simulink model "kalman_tank_based_fv"  (R2020b)
settings: Solver=ode45  StartTime=0.0  StopTime=30  RelTol=1e-3
values from neighbouring files (symbols this model uses):
  A = [1 Ts ... (first row only)    [kalman_hw7_main_fv.m]
  alpha = 0.5    [kalman_hw7_main_fv.m]
  Amp = 0.8    [kalman_hw7_main_fv.m]
  Be = 20    [kalman_hw7_main_fv.m]
  beta = 0.01    [kalman_hw7_main_fv.m]
  Bh = 1.5    [kalman_hw7_main_fv.m]
  Bs = 50    [kalman_hw7_main_fv.m]
  C = [1 0]    [kalman_hw7_main_fv.m]
  delay = 10    [kalman_hw7_main_fv.m]
  Dh = 2    [kalman_hw7_main_fv.m]
  Dm = 0    [kalman_hw7_main_fv.m]
  Ds = 0    [kalman_hw7_main_fv.m]
  Fc_lp = 5    [kalman_hw7_main_fv.m]
  Fc_sin = 0.1    [kalman_hw7_main_fv.m]
  H0_m = 1    [kalman_hw7_main_fv.m]
  H0_s = 1    [kalman_hw7_main_fv.m]
  H_D = 0.5    [kalman_hw7_main_fv.m]
  Je = 0    [kalman_hw7_main_fv.m]
  Jh = 0    [kalman_hw7_main_fv.m]
  Ke = 210    [kalman_hw7_main_fv.m]
  Kh = 0.1    [kalman_hw7_main_fv.m]
  Ks = 40    [kalman_hw7_main_fv.m]
  Mm = 0.5    [kalman_hw7_main_fv.m]
  Ms = 2    [kalman_hw7_main_fv.m]
  Ph = 1    [kalman_hw7_main_fv.m]
  posNoiseVar = 0.001    [kalman_hw7_main_fv.m]
  R_m = 1    [kalman_hw7_main_fv.m]
  R_s = 1    [kalman_hw7_main_fv.m]
  torqueNoiseVar = 0.001    [kalman_hw7_main_fv.m]
  Ts = 0.001    [kalman_hw7_main_fv.m]
  xe = 0.5    [kalman_hw7_main_fv.m]
undefined symbols (not defined in the file or in its folder): Discrete, Time
libraries: simulink x2, ctrlSharedLib x2
settings Model: Creator=nicol  LastModifiedBy=nicol

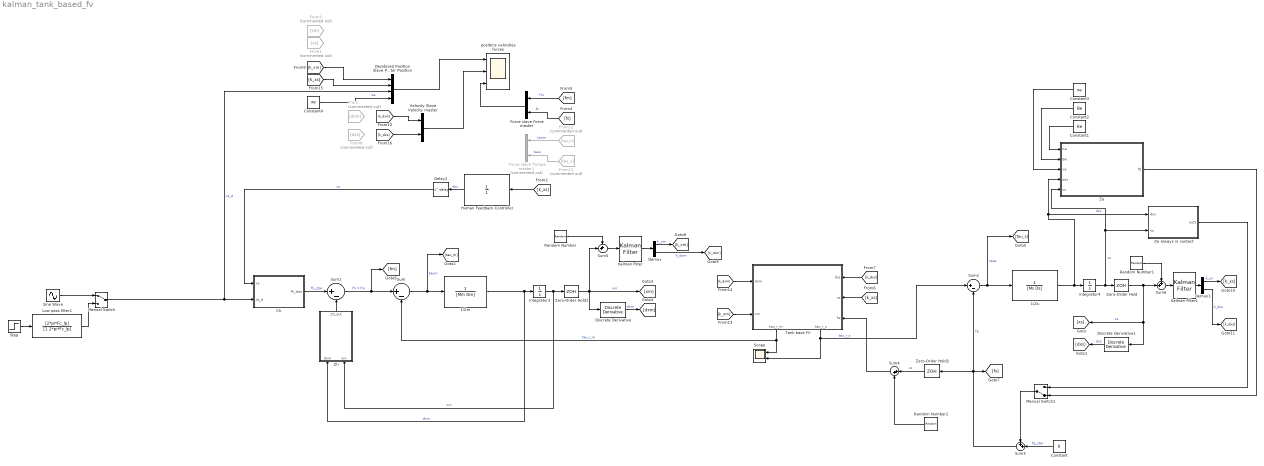
== system kalman_tank_based_fv ==
  1/Zm : TransferFcn  Denominator=[Mm Dm]
  1/Zs : TransferFcn  Denominator=[Ms Ds]
  Ch : Subsystem
  Constant : Constant  Value=0
  Constant1 : Constant  Value=Ke
  Constant2 : Constant  Value=Be
  Constant3 : Constant  Value=xe
  Constant4 : Constant  Value=xe
  Delay2 : Delay  DelayLength=delay  SampleTime=Ts
  Demux : Demux  Outputs=2
  Demux1 : Demux  Outputs=2
  Desidered Position Slave Position Master Position : Mux
  Discrete Derivative : simulink/Discrete/Discrete Derivative  gainval=1.0  ICPrevScaledInput=0.0  OutMin=[]  OutMax=[]  OutDataType=fixdt(1, 16)  OutScaling=2^-10  DoSatur=off
  Discrete Derivative1 : simulink/Discrete/Discrete Derivative  gainval=1.0  ICPrevScaledInput=0.0  OutMin=[]  OutMax=[]  OutDataType=fixdt(1, 16)  OutScaling=2^-10  DoSatur=off
  Force slave Force master : Mux  Inputs=2
  From : From  Commented=on  GotoTag=dxm
  From1 : From  Commented=on  GotoTag=xs
  From11 : From  Commented=on  GotoTag=tau_s
  From12 : From  Commented=on  GotoTag=tau_m
  From3 : From  Commented=on  GotoTag=xm
  From8 : From  Commented=on  GotoTag=dxs
  Human Feedback Controller : TransferFcn  Denominator=[1]
  Integrator3 : Integrator
  Integrator4 : Integrator
  Kalman Filter : ctrlSharedLib/Kalman Filter  TimeDomain=Discrete-Time  UseCurrentEstimator=on  ModelSource=Individual A, B, C, D matrices  ModelSourceVariable=ss(0.95,1,0,0,Ts)  A=A  B=1  C=C  D=0  NumberOfStates=1  NumberOfInputs=1  NumberOfOutputs=1  InitialEstimateSource=Dialog  X0=0  P0=10  UseK=off  UseGH=off  NumberOfProcessNoiseInputs=1  G=1  TimeInvariantG=on  H=0  TimeInvariantH=on  Q=Q_m  TimeInvariantQ=on  R=R_m  TimeInvariantR=on  N=0  TimeInvariantN=on  AddInputPort=off  AddEnablePort=off  OutputEstimatedY=off  OutputP=off  Ts=Ts
  Kalman Filter1 : ctrlSharedLib/Kalman Filter  TimeDomain=Discrete-Time  UseCurrentEstimator=on  ModelSource=Individual A, B, C, D matrices  ModelSourceVariable=ss(0.95,1,0,0,Ts)  A=A  B=1  C=C  D=0  NumberOfStates=1  NumberOfInputs=1  NumberOfOutputs=1  InitialEstimateSource=Dialog  X0=0  P0=10  UseK=off  UseGH=off  NumberOfProcessNoiseInputs=1  G=1  TimeInvariantG=on  H=0  TimeInvariantH=on  Q=Q_s  TimeInvariantQ=on  R=R_s  TimeInvariantR=on  N=0  TimeInvariantN=on  AddInputPort=off  AddEnablePort=off  OutputEstimatedY=off  OutputP=off  Ts=Ts
  Low pass filter1 : TransferFcn  Numerator=[2*pi*Fc_lp]  Denominator=[1 2*pi*Fc_lp]
  Manual Switch : ManualSwitch
  Manual Switch1 : ManualSwitch  CurrentSetting=0
  Random Number : RandomNumber  Variance=posNoiseVar  SampleTime=Ts
  Random Number1 : RandomNumber  Variance=posNoiseVar  SampleTime=Ts
  Random Number2 : RandomNumber  Variance=torqueNoiseVar  SampleTime=Ts
  Scope : Scope  NumInputPorts=2
  Sine Wave : Sin  Amplitude=Amp  Frequency=2*pi*Fc_sin  SampleTime=0
  Step : Step  Time=Amp  After=Amp  SampleTime=0
  Sum : Sum  Inputs=|+-
  Sum1 : Sum  Inputs=|+-
  Sum2 : Sum  Inputs=|+-
  Sum3 : Sum  Inputs=++|
  Sum4 : Sum  Inputs=|++
  Sum5 : Sum  Inputs=++|
  Sum6 : Sum  Inputs=++|
  Tank base FV : Subsystem
      settings: PortSchema="{\"entries\":[{\"content\":{\"sides\":[{\"content\":{\"connectorIds\":[\"In1\",\"In2\"]},\"type\":\"ConnectorPlacement.EquallySpacedRectSide\",\"uuid\":\"3a964002-fb37-4a92-b745-35f358b8e187\"},{\"content\":{\"connectorIds\":[\"In3\",\"In4\",\"In5\"],\"side\":\"RIGHT\"},\"type\":\"ConnectorPlacement.EquallySpacedRectSide\",\"uuid\":\"6a0ade08-0aa0-46a3-9e09-c310668c505c\"},{\"content\":{\"connectorIds\":[],\"side\":\"TOP\"},\"type\":\"ConnectorPlacement.EquallySpacedRectSide\",\"uuid\":\"1dfd7bbc-8185-4b5f-95de-42c58388ee02\"},{\"content\":{\"connectorIds\":[\"Out1\",\"Out2\"],\"side\":\"BOTTOM\"},\"type\":\"ConnectorPlacement.EquallySpacedRectSide\",\"uuid\":\"8c57ed43-4006-4572-ac50-c9adf88e8601\"},{\"content\":{\"connectorIds\":[],\"side\":\"HIDDEN\"},\"type\":\"ConnectorPlacement.EquallySpacedRectSide\",\"uuid\":\"15175a08-ca5b-4167-ba1d-f2e8cd3d814b\"}]},\"type\":\"ConnectorPlacement.EquallySpacedConnector\",\"uuid\":\"2bd1e993-3bc7-4875-9b20-3fb59092d5ec\"}],\"packageUris\":[\"http://schema.mathworks.com/mf0/Connector/R2020b\"],\"version\":\"1.0\"}"
  Torue slave Torque master1 : Mux  Commented=on  Inputs=2
  Velocity Slave Velocity master : Mux  Inputs=2
  Ze : MATLAB Function  TreatAsAtomicUnit=on
  Ze always in contact : Subsystem
  Zero-Order Hold : ZeroOrderHold  SampleTime=Ts
  Zero-Order Hold1 : ZeroOrderHold  SampleTime=Ts
  Zero-Order Hold2 : ZeroOrderHold  SampleTime=Ts
  Zh : Subsystem
  "positons velocities forces " : Scope  NumInputPorts=3
  wires:
  Ch/1(fh_star) -> Sum1/1  "fh_star"
  Zh/1(Zh_out) -> Sum1/2
  1/Zm/1 -> Zh/1(dxm), Integrator3/1  "dxm"
  Sum1/1 -> Sum/1, [fm]  "fh = fm"
  1/Zs/1 -> Integrator4/1, Ze always in contact/1(dxs), Ze/4(dxs)  "dxs"
  Sum2/1 -> 1/Zs/1, [tau_s]  "taus"
  Ze/1(fE) -> Manual Switch1/2
  Sum3/1 -> Zero-Order Hold2/1, Sum2/2, [fs]  "fe"
  Constant/1 -> Sum3/2  "fe_star"
  Constant1/1 -> Ze/1(Ke)
  Constant2/1 -> Ze/2(Be)
  Constant3/1 -> Ze/3(xe)
  Integrator4/1 -> Zero-Order Hold/1, Ze/5(xs), Ze always in contact/2(xs)  "xs"
  Manual Switch1/1 -> Sum3/1
  Ze always in contact/1(out1) -> Manual Switch1/1
  Sum/1 -> [tau_m], 1/Zm/1  "taum"
  Velocity Slave Velocity master/1 -> "positons velocities forces "/2
  Desidered Position Slave Position Master Position/1 -> "positons velocities forces "/1
  Manual Switch/1 -> Ch/2(xs_d), Desidered Position Slave Position Master Position/3  "xs_d"
  Integrator3/1 -> Zero-Order Hold1/1, Zh/2(xm)  "xm"
  [k_xs] -> Human Feedback Controller/1
  Delay2/1 -> Ch/1(xs)  "xs"
  Human Feedback Controller/1 -> Delay2/1  "dxs"
  Sine Wave/1 -> Manual Switch/1
  [k_dxm] -> Velocity Slave Velocity master/1
  [k_xs] -> Desidered Position Slave Position Master Position/2
  [k_xm] -> Desidered Position Slave Position Master Position/1
  Constant4/1 -> Desidered Position Slave Position Master Position/4  "xe"
  Step/1 -> Low pass filter1/1
  [k_dxs] -> Velocity Slave Velocity master/2
  Low pass filter1/1 -> Manual Switch/2
  Force slave Force master/1 -> "positons velocities forces "/3
  [fm] -> Force slave Force master/1  "fm"
  [fs] -> Force slave Force master/2  "fs"
  [k_dxm] -> Tank base FV/1(dxm)
  [k_xm] -> Tank base FV/2(xm)
  [k_dxs] -> Tank base FV/3(dxs)
  [k_xs] -> Tank base FV/4(xs)
  Tank base FV/1(tau_r_m) -> Sum/2, Scope/1  "tau_r_m"
  Tank base FV/2(tau_r_s) -> Sum2/1, Scope/2  "tau_r_s"
  From12/1 -> Torue slave Torque master1/1  "taum"
  From11/1 -> Torue slave Torque master1/2  "taus"
  Zero-Order Hold2/1 -> Sum4/1  "xs"
  Sum5/1 -> Kalman Filter/1
  Demux/1 -> [k_xm]  "k_xm"
  Random Number/1 -> Sum5/1
  Zero-Order Hold1/1 -> Discrete Derivative/1, Sum5/2, [xm]  "xm"
  Discrete Derivative/1 -> [dxm]  "dxm"
  Kalman Filter/1 -> Demux/1
  Demux/2 -> [k_dxm]  "k_dxm"
  Demux1/2 -> [k_dxs]  "k_dxs"
  Demux1/1 -> [k_xs]  "k_xs"
  Sum6/1 -> Kalman Filter1/1
  Kalman Filter1/1 -> Demux1/1
  Random Number1/1 -> Sum6/1
  Zero-Order Hold/1 -> Sum6/2, [xs], Discrete Derivative1/1  "xs"
  Discrete Derivative1/1 -> [dxs]  "dxs"
  Random Number2/1 -> Sum4/2
  Sum4/1 -> Tank base FV/5(fe)

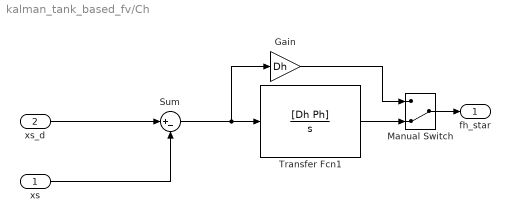
== system kalman_tank_based_fv/Ch ==
  xs : Inport
  xs_d : Inport  Port=2
  Gain : Gain  Gain=Dh
  Manual Switch : ManualSwitch  CurrentSetting=0
  Sum : Sum  Inputs=|+-
  Transfer Fcn1 : TransferFcn  Numerator=[Dh Ph]  Denominator=[1 0]
  fh_star : Outport
  wires:
  xs/1 -> Sum/2
  Sum/1 -> Gain/1, Transfer Fcn1/1
  xs_d/1 -> Sum/1
  Transfer Fcn1/1 -> Manual Switch/2
  Manual Switch/1 -> fh_star/1
  Gain/1 -> Manual Switch/1

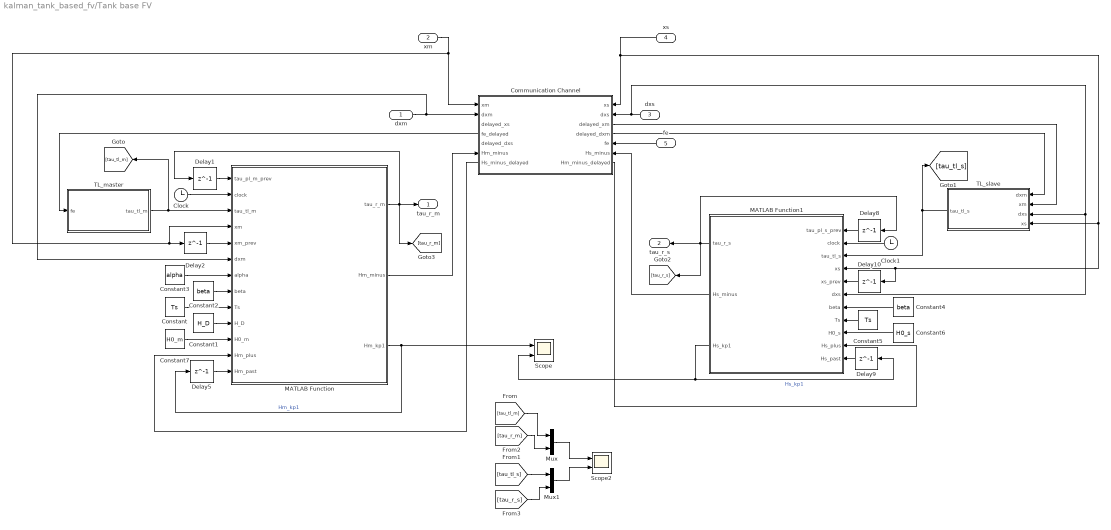
== system kalman_tank_based_fv/Tank base FV ==
  dxm : Inport
  xm : Inport  Port=2
  dxs : Inport  Port=3
  xs : Inport  Port=4
  fe : Inport  Port=5
  Clock : Clock
  Clock1 : Clock
  Communication Channel : Subsystem
      settings: PortSchema="{\"entries\":[{\"content\":{\"sides\":[{\"content\":{\"connectorIds\":[\"In1\",\"In2\",\"Out5\",\"Out6\",\"In3\",\"In4\",\"Out7\"]},\"type\":\"ConnectorPlacement.EquallySpacedRectSide\",\"uuid\":\"707b854d-ad7a-498f-bed1-9a4f8657ce88\"},{\"content\":{\"connectorIds\":[\"In5\",\"In6\",\"Out1\",\"Out2\",\"Out3\",\"In7\",\"Out4\"],\"side\":\"RIGHT\"},\"type\":\"ConnectorPlacement.EquallySpacedRectSide\",\"uuid\":\"12f3e034-857d-4081-a3d0-204c7e32b1d7\"},{\"content\":{\"connectorIds\":[],\"side\":\"TOP\"},\"type\":\"ConnectorPlacement.EquallySpacedRectSide\",\"uuid\":\"fb6b09f7-6084-4258-a6c2-180f375b33c2\"},{\"content\":{\"connectorIds\":[],\"side\":\"HIDDEN\"},\"type\":\"ConnectorPlacement.EquallySpacedRectSide\",\"uuid\":\"424096ec-dcd8-463d-bba6-855fd00452bd\"}]},\"type\":\"ConnectorPlacement.EquallySpacedConnector\",\"uuid\":\"13b09cb8-9f61-41a9-b654-31f5f7de73c5\"}],\"packageUris\":[\"http://schema.mathworks.com/mf0/Connector/R2020b\"],\"version\":\"1.0\"}"
  Constant : Constant  Value=Ts
  Constant1 : Constant  Value=H_D
  Constant2 : Constant  Value=beta
  Constant3 : Constant  Value=alpha
  Constant4 : Constant  Value=beta
  Constant5 : Constant  Value=Ts
  Constant6 : Constant  Value=H0_s
  Constant7 : Constant  Value=H0_m
  Delay{1..2,5,8..10} (6 alike) : Delay  DelayLength=1
  MATLAB Function : MATLAB Function  TreatAsAtomicUnit=on
  MATLAB Function1 : MATLAB Function  TreatAsAtomicUnit=on
  Mux : Mux  Inputs=2
  Mux1 : Mux  Inputs=2
  Scope : Scope  NumInputPorts=2
  Scope2 : Scope  NumInputPorts=2
  TL_master : Subsystem
  TL_slave : Subsystem
  tau_r_m : Outport
  tau_r_s : Outport  Port=2
  wires:
  TL_master/1(tau_tl_m) -> [tau_tl_m], MATLAB Function/3(tau_tl_m)
  Clock/1 -> MATLAB Function/2(clock)
  MATLAB Function/1(tau_r_m) -> [tau_r_m], Delay1/1, tau_r_m/1
  Delay1/1 -> MATLAB Function/1(tau_pl_m_prev)
  Delay2/1 -> MATLAB Function/5(xm_prev)
  Delay5/1 -> MATLAB Function/13(Hm_past)
  Constant/1 -> MATLAB Function/9(Ts)
  Constant1/1 -> MATLAB Function/10(H_D)
  MATLAB Function/3(Hm_kp1) -> Delay5/1, Scope/1  "Hm_kp1"
  Constant2/1 -> MATLAB Function/8(beta)
  Constant3/1 -> MATLAB Function/7(alpha)
  Communication Channel/4(Hs_minus_delayed) -> MATLAB Function/12(Hm_plus)
  MATLAB Function1/1(tau_r_s) -> Delay8/1, [tau_r_s], tau_r_s/1
  Delay8/1 -> MATLAB Function1/1(tau_pl_s_prev)
  Clock1/1 -> MATLAB Function1/2(clock)
  Constant4/1 -> MATLAB Function1/7(beta)
  Constant5/1 -> MATLAB Function1/8(Ts)
  Delay9/1 -> MATLAB Function1/11(Hs_past)
  MATLAB Function1/3(Hs_kp1) -> Scope/2, Delay9/1  "Hs_kp1"
  Delay10/1 -> MATLAB Function1/5(xs_prev)
  xs/1 -> Communication Channel/1(xs), Delay10/1, MATLAB Function1/4(xs), TL_slave/4(xs)
  xm/1 -> Communication Channel/5(xm), MATLAB Function/4(xm), Delay2/1
  dxm/1 -> MATLAB Function/6(dxm), Communication Channel/6(dxm)
  dxs/1 -> MATLAB Function1/6(dxs), TL_slave/3(dxs), Communication Channel/2(dxs)
  MATLAB Function/2(Hm_minus) -> Communication Channel/7(Hm_minus)
  MATLAB Function1/2(Hs_minus) -> Communication Channel/4(Hs_minus)
  Communication Channel/7(Hm_minus_delayed) -> MATLAB Function1/10(Hs_plus)
  Communication Channel/5(delayed_xm) -> TL_slave/2(xm)
  Communication Channel/6(delayed_dxm) -> TL_slave/1(dxm)
  TL_slave/1(tau_tl_s) -> [tau_tl_s], MATLAB Function1/3(tau_tl_s)
  [tau_tl_m] -> Mux/1
  [tau_tl_s] -> Mux1/1
  [tau_r_m] -> Mux/2
  [tau_r_s] -> Mux1/2
  Mux/1 -> Scope2/1
  Mux1/1 -> Scope2/2
  fe/1 -> Communication Channel/3(fe)
  Communication Channel/2(fe_delayed) -> TL_master/1(fe)
  Constant6/1 -> MATLAB Function1/9(H0_s)
  Constant7/1 -> MATLAB Function/11(H0_m)

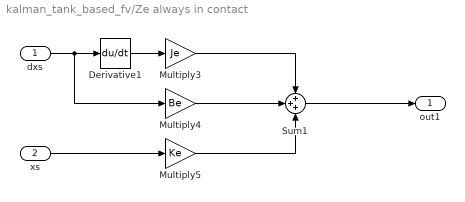
== system kalman_tank_based_fv/Ze always in contact ==
  dxs : Inport
  xs : Inport  Port=2
  Derivative1 : Derivative
  Multiply3 : Gain  Gain=Je
  Multiply4 : Gain  Gain=Be
  Multiply5 : Gain  Gain=Ke
  Sum1 : Sum  Inputs=+++
  out1 : Outport
  wires:
  Sum1/1 -> out1/1
  Multiply4/1 -> Sum1/2
  Multiply5/1 -> Sum1/3
  dxs/1 -> Multiply4/1, Derivative1/1
  Derivative1/1 -> Multiply3/1
  xs/1 -> Multiply5/1
  Multiply3/1 -> Sum1/1

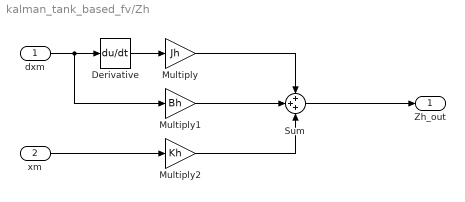
== system kalman_tank_based_fv/Zh ==
  dxm : Inport
  xm : Inport  Port=2
  Derivative : Derivative
  Multiply : Gain  Gain=Jh
  Multiply1 : Gain  Gain=Bh
  Multiply2 : Gain  Gain=Kh
  Sum : Sum  Inputs=+++
  Zh_out : Outport
  wires:
  dxm/1 -> Multiply1/1, Derivative/1
  Derivative/1 -> Multiply/1
  Sum/1 -> Zh_out/1
  xm/1 -> Multiply2/1
  Multiply1/1 -> Sum/2
  Multiply/1 -> Sum/1
  Multiply2/1 -> Sum/3

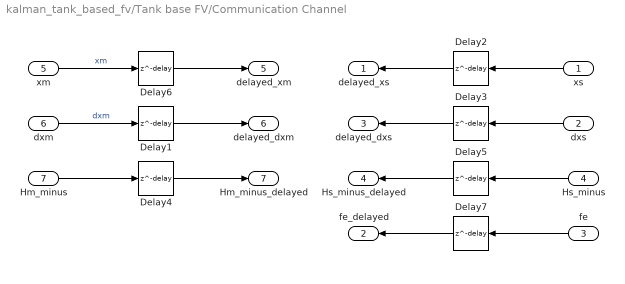
== system kalman_tank_based_fv/Tank base FV/Communication Channel ==
  xs : Inport
  dxs : Inport  Port=2
  fe : Inport  Port=3
  Hs_minus : Inport  Port=4
  xm : Inport  Port=5
  dxm : Inport  Port=6
  Hm_minus : Inport  Port=7
  Delay{1..7} (7 alike) : Delay  DelayLength=delay  SampleTime=Ts
  delayed_xs : Outport
  fe_delayed : Outport  Port=2
  delayed_dxs : Outport  Port=3
  Hs_minus_delayed : Outport  Port=4
  delayed_xm : Outport  Port=5
  delayed_dxm : Outport  Port=6
  Hm_minus_delayed : Outport  Port=7
  wires:
  xm/1 -> Delay6/1  "xm"
  dxm/1 -> Delay1/1  "dxm"
  Delay6/1 -> delayed_xm/1
  Delay1/1 -> delayed_dxm/1
  Delay3/1 -> delayed_dxs/1
  xs/1 -> Delay2/1
  dxs/1 -> Delay3/1
  Delay2/1 -> delayed_xs/1
  Hm_minus/1 -> Delay4/1
  Delay4/1 -> Hm_minus_delayed/1
  Delay5/1 -> Hs_minus_delayed/1
  Hs_minus/1 -> Delay5/1
  fe/1 -> Delay7/1
  Delay7/1 -> fe_delayed/1

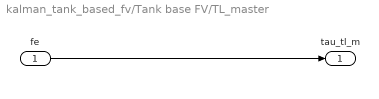
== system kalman_tank_based_fv/Tank base FV/TL_master ==
  fe : Inport
  tau_tl_m : Outport
  wires:
  fe/1 -> tau_tl_m/1

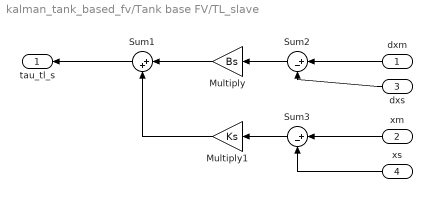
== system kalman_tank_based_fv/Tank base FV/TL_slave ==
  dxm : Inport
  xm : Inport  Port=2
  dxs : Inport  Port=3
  xs : Inport  Port=4
  Multiply : Gain  Gain=Bs
  Multiply1 : Gain  Gain=Ks
  Sum1 : Sum  Inputs=|++
  Sum2 : Sum  Inputs=|+-
  Sum3 : Sum  Inputs=|+-
  tau_tl_s : Outport
  wires:
  Sum2/1 -> Multiply/1
  Multiply1/1 -> Sum1/2
  Multiply/1 -> Sum1/1
  Sum1/1 -> tau_tl_s/1
  Sum3/1 -> Multiply1/1
  xs/1 -> Sum3/2
  dxs/1 -> Sum2/2
  xm/1 -> Sum3/1
  dxm/1 -> Sum2/1

== matlab function kalman_tank_based_fv/Tank base FV/MATLAB Function ==
  data: tau_pl_m_prev input; clock input; tau_r_m output; Hm_minus output; tau_tl_m input; xm input; xm_prev input; dxm input; alpha input; beta input; Ts input; H_D input; H0_m input; Hm_plus input; Hm_past input; Hm_kp1 output
function [tau_r_m, Hm_minus, Hm_kp1] = passivity_layer_master(tau_pl_m_prev, clock, tau_tl_m, xm, xm_prev, dxm, alpha, beta, Ts, H_D, H0_m, Hm_plus, Hm_past)
    if clock == 0
        Hm_past = H0_m;
        tau_pl_m_prev = 0;
        xm_prev = 0; 
    end
    
    delta_xm = xm - xm_prev;
    delta_H_used = tau_pl_m_prev*(delta_xm);
    Hm_k = Hm_past + Hm_plus - delta_H_used;

    
    % Computation of H_kp1
    
    % Send energy
    if (Hm_k > 0)
        Hm_minus =  beta*Hm_k;
        Hm_kp1 = Hm_k - Hm_minus;  
    else
        Hm_minus = 0;
        Hm_kp1 = 0;
    end
    
    % TLC check
    if(Hm_kp1 < H_D)
       d = alpha*(H_D - Hm_kp1);
       tau_TLC = -d*dxm;
    else
       tau_TLC = 0;
    end
    
    % Compute tau limits
    if Hm_kp1 <= 0 
        tau_max_m_1 = 0;
    else
        tau_max_m_1 = tau_tl_m;
    end
    
    if abs(dxm) < 0.001
        tau_max_m_2 = 1e3;
    else
        tau_max_m_2 =  Hm_kp1/(dxm*Ts);
    end
    
    tau_pl_m = sign(tau_tl_m)*min([abs(tau_tl_m), abs(tau_max_m_1), abs(tau_max_m_2)]);
    
    tau_r_m = tau_pl_m + tau_TLC;

end

== matlab function kalman_tank_based_fv/Ze ==
  data: Ke input; fE output; Be input; xe input; dxs input; xs input
function fE = environment(Ke, Be, xe, dxs, xs)
if(xs > xe)
    fE = Ke*(xs - xe) + Be*dxs;
else
    fE=0;
end

== matlab function kalman_tank_based_fv/Tank base FV/MATLAB Function1 ==
  data: tau_r_s output; Hs_minus output; tau_pl_s_prev input; Hs_kp1 output; clock input; tau_tl_s input; xs input; xs_prev input; dxs input; beta input; Ts input; H0_s input; Hs_plus input; Hs_past input
function [tau_r_s, Hs_minus, Hs_kp1 ] = passivity_layer_slave(tau_pl_s_prev, clock, tau_tl_s, xs, xs_prev, dxs, beta, Ts, H0_s, Hs_plus, Hs_past)
    if clock == 0
        Hs_past = H0_s;
        tau_pl_s_prev = 0;
        xs_prev = 0;
    end
    
    delta_xs = xs - xs_prev;
    delta_H_used = tau_pl_s_prev*(delta_xs);
    Hs_k = Hs_past + Hs_plus - delta_H_used;
 
    % Send energy
    if (Hs_k > 0)
        Hs_minus =  beta*Hs_k;
        Hs_kp1 = Hs_k - Hs_minus;  
    else
        Hs_kp1 = 0;
        Hs_minus = 0;
    end
    
    % Compute tau limits
    if Hs_kp1 <= 0 
        tau_max_s_1 = 0;
    else
        tau_max_s_1 = tau_tl_s;
    end
    
    if abs(dxs) < 0.001
        tau_max_s_2 = 1e3;
    else
        tau_max_s_2 =  Hs_kp1/(dxs*Ts);
    end
    
    tau_pl_s = sign(tau_tl_s)*min([abs(tau_tl_s), abs(tau_max_s_1), abs(tau_max_s_2)]);
    
    tau_r_s = tau_pl_s;
    
   
end
